simulink model "task2_8"  (R2021a)
settings: Solver=VariableStepAuto  StartTime=0.0  StopTime=10.0  RelTol=1e-3
libraries: simulink x2
settings Model: Creator=reemb  LastModifiedBy=reemb

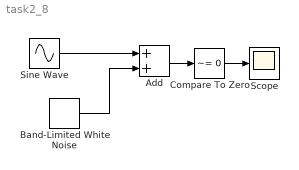
== system task2_8 ==
  Add : Sum
  Band-Limited White Noise : simulink/Sources/Band-Limited White Noise  Cov=[0.1]  Ts=0.1  seed=[23341]
  Compare To Zero : simulink/Logic and Bit Operations/Compare To Zero  relop=~=  OutDataTypeStr=boolean
  Scope : Scope
  Sine Wave : Sin  SampleTime=0
  wires:
  Compare To Zero/1 -> Scope/1
  Add/1 -> Compare To Zero/1
  Sine Wave/1 -> Add/1
  Band-Limited White Noise/1 -> Add/2
